simulink model "simple_AC"  (R2016a)
settings: Solver=VariableStepAuto  StartTime=0.0  StopTime=50  RelTol=1e-3
settings Model: Creator=Priscilla  LastModifiedBy=Priscilla

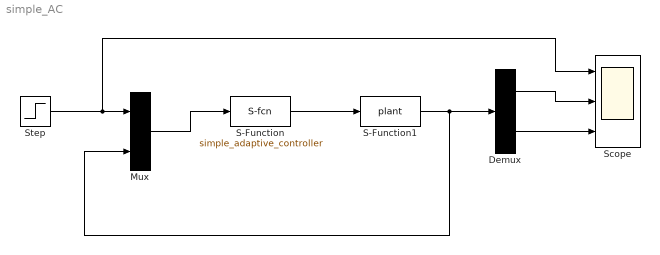
== system simple_AC ==
  Demux : Demux  Outputs=2
  Mux : Mux  Inputs=2
  S-Function : S-Function  FunctionName=simple_adaptive_controller  SFunctionDeploymentMode=off  EnableBusSupport=off
  S-Function1 : S-Function  FunctionName=plant  SFunctionDeploymentMode=off  EnableBusSupport=off
  Scope : Scope  NumInputPorts=3
  Step : Step  SampleTime=0
  wires:
  S-Function/1 -> S-Function1/1
  Demux/1 -> Scope/2
  Step/1 -> Mux/1, Scope/1
  Mux/1 -> S-Function/1
  Demux/2 -> Scope/3
  S-Function1/1 -> Mux/2, Demux/1
